simulink model "xaui_monitor_test"  (Simulink 7.0)
settings: Solver=ode45  StartTime=0.0  StopTime=100  RelTol=1e-3
libraries: xbsIndex_r4 x34, casper_library_misc x5
settings Model: Creator=mdexter  LastModifiedBy=mdexter

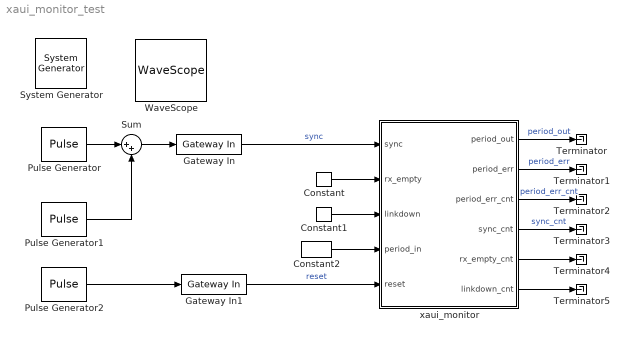
== system xaui_monitor_test ==
  " System Generator" : xbsIndex_r4/ System Generator  Tag=genX  SystemSampleTime=-1  xilinxfamily=Virtex4  part=xc4vsx35  speed=-10  package=ff668  synthesis_tool=XST  clock_wrapper=Clock Enables  directory=./netlist  testbench=off  simulink_period=1  sysclk_period=100  dcm_input_clock_period=100  incr_netlist=off  trim_vbits=Everywhere in SubSystem  dbl_ovrd=According to Block Masks  core_generation=According to Block Masks  run_coregen=off  deprecated_control=off  eval_field=0  block_type=sysgen
      settings: block_version=10.1.3
  Constant : xbsIndex_r4/Constant  arith_type=Boolean  const=0  n_bits=16  bin_pt=14  explicit_period=on  period=1  equ=P=C  opselect=C  inp2=PCIN>>17  opr=+  inp1=P  carry=CIN  dbl_ovrd=off  block_type=constant
  Constant1 : xbsIndex_r4/Constant  arith_type=Boolean  const=0  n_bits=16  bin_pt=14  explicit_period=on  period=1  equ=P=C  opselect=C  inp2=PCIN>>17  opr=+  inp1=P  carry=CIN  dbl_ovrd=off  block_type=constant
  Constant2 : xbsIndex_r4/Constant  arith_type=Unsigned  const=10  n_bits=32  bin_pt=0  explicit_period=on  period=1  equ=P=C  opselect=C  inp2=PCIN>>17  opr=+  inp1=P  carry=CIN  dbl_ovrd=off  block_type=constant
  Gateway In : xbsIndex_r4/Gateway In  arith_type=Boolean  n_bits=16  bin_pt=14  quantization="Round  (unbiased: +/- Inf)"  overflow=Saturate  period=1  dbl_ovrd=off  timing_constraint=None  locs_specified=off  LOCs={}  block_type=gatewayin
      settings: infoedit="Gateway in block.  Converts inputs of type Simulink integer, double and fixed point to  Xilinx fixed point type.<P><P>Hardware notes:  In hardware these blocks become top level input ports."  block_version=10.1.3
  Gateway In1 : xbsIndex_r4/Gateway In  arith_type=Boolean  n_bits=16  bin_pt=14  quantization="Round  (unbiased: +/- Inf)"  overflow=Saturate  period=1  dbl_ovrd=off  timing_constraint=None  locs_specified=off  LOCs={}  block_type=gatewayin
      settings: infoedit="Gateway in block.  Converts inputs of type Simulink integer, double and fixed point to  Xilinx fixed point type.<P><P>Hardware notes:  In hardware these blocks become top level input ports."  block_version=10.1.3
  Pulse Generator : DiscretePulseGenerator  Period=10  VectorParams1D=off
  Pulse Generator1 : DiscretePulseGenerator  Period=1e3  PhaseDelay=34  VectorParams1D=off
  Pulse Generator2 : DiscretePulseGenerator  Period=1e3  PhaseDelay=49  VectorParams1D=off
  Sum : Sum  Inputs=|++  OutDataType=sfix(16)  OutScaling=2^0
  Terminator{,1..5} (6 alike) : Terminator
  WaveScope : xbsIndex_r4/WaveScope  block_type=wavescope
      settings: block_version=10.1.3
  xaui_monitor : Subsystem
  wires:
  Gateway In/1 -> xaui_monitor/1(sync)  "sync"
  Constant/1 -> xaui_monitor/2(rx_empty)
  Constant1/1 -> xaui_monitor/3(linkdown)
  Constant2/1 -> xaui_monitor/4(period_in)
  Gateway In1/1 -> xaui_monitor/5(reset)  "reset"
  xaui_monitor/1(period_out) -> Terminator/1  "period_out"
  xaui_monitor/2(period_err) -> Terminator1/1  "period_err"
  xaui_monitor/3(period_err_cnt) -> Terminator2/1  "period_err_cnt"
  xaui_monitor/4(sync_cnt) -> Terminator3/1  "sync_cnt"
  xaui_monitor/5(rx_empty_cnt) -> Terminator4/1
  xaui_monitor/6(linkdown_cnt) -> Terminator5/1
  Pulse Generator/1 -> Sum/1
  Sum/1 -> Gateway In/1
  Pulse Generator1/1 -> Sum/2
  Pulse Generator2/1 -> Gateway In1/1

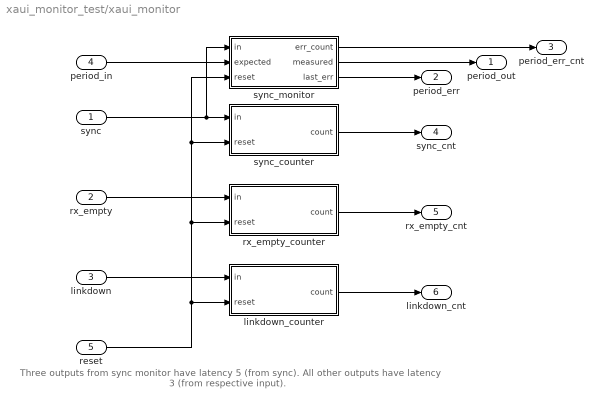
== system xaui_monitor_test/xaui_monitor ==
  note: Three outputs from sync monitor have latency 5 (from sync).
      | All other outputs have latency 3 (from respective input).
  sync : Inport
  rx_empty : Inport  Port=2
  linkdown : Inport  Port=3
  period_in : Inport  Port=4
  reset : Inport  Port=5
  linkdown_counter : Subsystem
      settings: AttributesFormatString=rising
  rx_empty_counter : Subsystem
      settings: AttributesFormatString=rising
  sync_counter : Subsystem
      settings: AttributesFormatString=rising
  sync_monitor : Subsystem
  period_out : Outport
  period_err : Outport  Port=2
  period_err_cnt : Outport  Port=3
  sync_cnt : Outport  Port=4
  rx_empty_cnt : Outport  Port=5
  linkdown_cnt : Outport  Port=6
  wires:
  sync/1 -> sync_monitor/1(in), sync_counter/1(in)
  sync_monitor/1(err_count) -> period_err_cnt/1
  period_in/1 -> sync_monitor/2(expected)
  sync_monitor/2(measured) -> period_out/1
  sync_monitor/3(last_err) -> period_err/1
  sync_counter/1(count) -> sync_cnt/1
  rx_empty/1 -> rx_empty_counter/1(in)
  rx_empty_counter/1(count) -> rx_empty_cnt/1
  linkdown/1 -> linkdown_counter/1(in)
  linkdown_counter/1(count) -> linkdown_cnt/1
  reset/1 -> sync_monitor/3(reset), sync_counter/2(reset), rx_empty_counter/2(reset), linkdown_counter/2(reset)

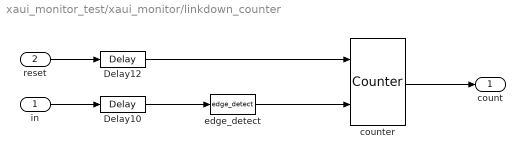
== system xaui_monitor_test/xaui_monitor/linkdown_counter ==
  in : Inport  OutDataType=sfix(16)  OutScaling=2^0
  reset : Inport  Port=2  OutDataType=sfix(16)  OutScaling=2^0
  Delay10 : xbsIndex_r4/Delay  en=off  latency=1  dbl_ovrd=off  reg_retiming=off  block_type=delay
      settings: xl_area=[0, 0, 0, 0, 0, 0, 0]
  Delay12 : xbsIndex_r4/Delay  en=off  latency=1  dbl_ovrd=off  reg_retiming=off  block_type=delay
      settings: xl_area=[0, 0, 0, 0, 0, 0, 0]
  counter : xbsIndex_r4/Counter  cnt_type=Free Running  cnt_to=Inf  operation=Up  start_count=0  cnt_by_val=1  arith_type=Unsigned  n_bits=32  bin_pt=0  load_pin=off  rst=on  en=on  explicit_period=off  period=1  dbl_ovrd=off  use_behavioral_HDL=on  use_rpm=on  implementation=Fabric  block_type=counter
      settings: xl_area=[0, 0, 0, 0, 0, 0, 0]
  edge_detect : casper_library_misc/edge_detect  SystemSampleTime=-1  edge=Rising  polarity=Active High  x_in=[0 0.08 0.08 0.16 0.16 0.24 0.24 0.32 0.32 0.4]  y_in="[-1 -1  1  1  1  1  1  1  1  1]"  x_out=[0.6 0.68 0.68 0.76 0.76 0.84 0.84 0.92 0.92 1]  y_out="[-1 -1  1  1 -1 -1 -1 -1 -1 -1]"
  count : Outport  OutDataType=sfix(16)  OutScaling=2^0
  wires:
  in/1 -> Delay10/1
  reset/1 -> Delay12/1
  Delay10/1 -> edge_detect/1
  Delay12/1 -> counter/1
  counter/1 -> count/1
  edge_detect/1 -> counter/2

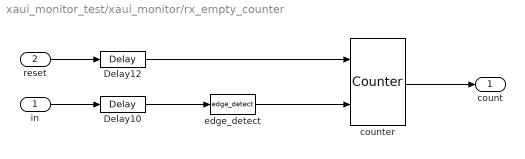
== system xaui_monitor_test/xaui_monitor/rx_empty_counter ==
  in : Inport  OutDataType=sfix(16)  OutScaling=2^0
  reset : Inport  Port=2  OutDataType=sfix(16)  OutScaling=2^0
  Delay10 : xbsIndex_r4/Delay  en=off  latency=1  dbl_ovrd=off  reg_retiming=off  block_type=delay
      settings: xl_area=[0, 0, 0, 0, 0, 0, 0]
  Delay12 : xbsIndex_r4/Delay  en=off  latency=1  dbl_ovrd=off  reg_retiming=off  block_type=delay
      settings: xl_area=[0, 0, 0, 0, 0, 0, 0]
  counter : xbsIndex_r4/Counter  cnt_type=Free Running  cnt_to=Inf  operation=Up  start_count=0  cnt_by_val=1  arith_type=Unsigned  n_bits=32  bin_pt=0  load_pin=off  rst=on  en=on  explicit_period=off  period=1  dbl_ovrd=off  use_behavioral_HDL=on  use_rpm=on  implementation=Fabric  block_type=counter
      settings: xl_area=[0, 0, 0, 0, 0, 0, 0]
  edge_detect : casper_library_misc/edge_detect  SystemSampleTime=-1  edge=Rising  polarity=Active High  x_in=[0 0.08 0.08 0.16 0.16 0.24 0.24 0.32 0.32 0.4]  y_in="[-1 -1  1  1  1  1  1  1  1  1]"  x_out=[0.6 0.68 0.68 0.76 0.76 0.84 0.84 0.92 0.92 1]  y_out="[-1 -1  1  1 -1 -1 -1 -1 -1 -1]"
  count : Outport  OutDataType=sfix(16)  OutScaling=2^0
  wires:
  in/1 -> Delay10/1
  reset/1 -> Delay12/1
  Delay10/1 -> edge_detect/1
  Delay12/1 -> counter/1
  counter/1 -> count/1
  edge_detect/1 -> counter/2

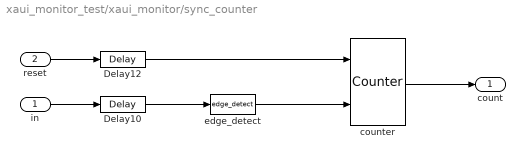
== system xaui_monitor_test/xaui_monitor/sync_counter ==
  in : Inport  OutDataType=sfix(16)  OutScaling=2^0
  reset : Inport  Port=2  OutDataType=sfix(16)  OutScaling=2^0
  Delay10 : xbsIndex_r4/Delay  en=off  latency=1  dbl_ovrd=off  reg_retiming=off  block_type=delay
      settings: xl_area=[0, 0, 0, 0, 0, 0, 0]
  Delay12 : xbsIndex_r4/Delay  en=off  latency=1  dbl_ovrd=off  reg_retiming=off  block_type=delay
      settings: xl_area=[0, 0, 0, 0, 0, 0, 0]
  counter : xbsIndex_r4/Counter  cnt_type=Free Running  cnt_to=Inf  operation=Up  start_count=0  cnt_by_val=1  arith_type=Unsigned  n_bits=32  bin_pt=0  load_pin=off  rst=on  en=on  explicit_period=off  period=1  dbl_ovrd=off  use_behavioral_HDL=on  use_rpm=on  implementation=Fabric  block_type=counter
      settings: xl_area=[0, 0, 0, 0, 0, 0, 0]
  edge_detect : casper_library_misc/edge_detect  SystemSampleTime=-1  edge=Rising  polarity=Active High  x_in=[0 0.08 0.08 0.16 0.16 0.24 0.24 0.32 0.32 0.4]  y_in="[-1 -1  1  1  1  1  1  1  1  1]"  x_out=[0.6 0.68 0.68 0.76 0.76 0.84 0.84 0.92 0.92 1]  y_out="[-1 -1  1  1 -1 -1 -1 -1 -1 -1]"
  count : Outport  OutDataType=sfix(16)  OutScaling=2^0
  wires:
  in/1 -> Delay10/1
  reset/1 -> Delay12/1
  Delay10/1 -> edge_detect/1
  Delay12/1 -> counter/1
  counter/1 -> count/1
  edge_detect/1 -> counter/2

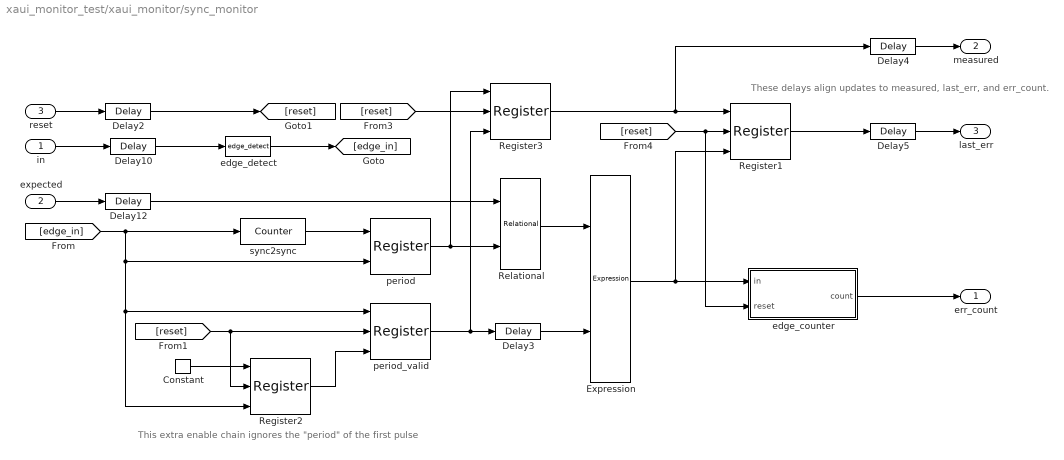
== system xaui_monitor_test/xaui_monitor/sync_monitor ==
  note: This extra enable chain ignores the "period" of the first pulse
  note: These delays align updates to
      | measured, last_err, and err_count.
  in : Inport
  expected : Inport  Port=2
  reset : Inport  Port=3
  Constant : xbsIndex_r4/Constant  arith_type=Boolean  const=1  n_bits=16  bin_pt=14  explicit_period=on  period=1  equ=P=C  opselect=C  inp2=PCIN>>17  opr=+  inp1=P  carry=CIN  dbl_ovrd=off  block_type=constant
  Delay{2..3,5,10,12} (5 alike) : xbsIndex_r4/Delay  en=off  latency=1  dbl_ovrd=off  reg_retiming=off  block_type=delay
      settings: xl_area=[0, 0, 0, 0, 0, 0, 0]
  Delay4 : xbsIndex_r4/Delay  en=off  latency=2  dbl_ovrd=off  reg_retiming=off  block_type=delay
      settings: xl_area=[0, 0, 0, 0, 0, 0, 0]
  Expression : xbsIndex_r4/Expression  expression=a & b  align_bp=on  en=off  latency=0  precision=Full  arith_type=Unsigned  n_bits=16  bin_pt=0  dbl_ovrd=off  block_type=expr
      settings: block_version=10.1.3
  Register1 : xbsIndex_r4/Register  init=0  rst=on  en=on  dbl_ovrd=off  block_type=register
  Register2 : xbsIndex_r4/Register  init=0  rst=on  en=on  dbl_ovrd=off  block_type=register
  Register3 : xbsIndex_r4/Register  init=0  rst=on  en=on  dbl_ovrd=off  block_type=register
  Relational : xbsIndex_r4/Relational  mode=a!=b  en=off  latency=1  dbl_ovrd=off  block_type=relational
      settings: block_version=10.1.3
  edge_counter : Subsystem
      settings: AttributesFormatString=rising
  edge_detect : casper_library_misc/edge_detect  SystemSampleTime=-1  edge=Rising  polarity=Active High  x_in=[0 0.08 0.08 0.16 0.16 0.24 0.24 0.32 0.32 0.4]  y_in="[-1 -1  1  1  1  1  1  1  1  1]"  x_out=[0.6 0.68 0.68 0.76 0.76 0.84 0.84 0.92 0.92 1]  y_out="[-1 -1  1  1 -1 -1 -1 -1 -1 -1]"
  period : xbsIndex_r4/Register  init=0  rst=off  en=on  dbl_ovrd=off  block_type=register
  period_valid : xbsIndex_r4/Register  init=0  rst=on  en=on  dbl_ovrd=off  block_type=register
  sync2sync : xbsIndex_r4/Counter  cnt_type=Free Running  cnt_to=Inf  operation=Up  start_count=1  cnt_by_val=1  arith_type=Unsigned  n_bits=32  bin_pt=0  load_pin=off  rst=on  en=off  explicit_period=off  period=1  dbl_ovrd=off  use_behavioral_HDL=on  use_rpm=on  implementation=Fabric  block_type=counter
      settings: xl_area=[0, 0, 0, 0, 0, 0, 0]
  err_count : Outport  OutDataType=sfix(16)  OutScaling=2^0
  measured : Outport  Port=2  OutDataType=sfix(16)  OutScaling=2^0
  last_err : Outport  Port=3  OutDataType=sfix(16)  OutScaling=2^0
  wires:
  sync2sync/1 -> period/1
  [edge_in] -> sync2sync/1, period/2, period_valid/1, Register2/3
  Relational/1 -> Expression/1
  Delay3/1 -> Expression/2
  Expression/1 -> edge_counter/1(in), Register1/3
  period/1 -> Relational/2, Register3/1
  expected/1 -> Delay12/1
  reset/1 -> Delay2/1
  edge_counter/1(count) -> err_count/1
  Register1/1 -> Delay5/1
  Register3/1 -> Register1/1, Delay4/1
  Delay10/1 -> edge_detect/1
  in/1 -> Delay10/1
  Delay12/1 -> Relational/1
  edge_detect/1 -> [edge_in]
  Delay2/1 -> [reset]
  Constant/1 -> Register2/1
  period_valid/1 -> Delay3/1, Register3/3
  Delay4/1 -> measured/1
  Delay5/1 -> last_err/1
  Register2/1 -> period_valid/3
  [reset] -> period_valid/2, Register2/2
  [reset] -> Register3/2
  [reset] -> Register1/2, edge_counter/2(reset)

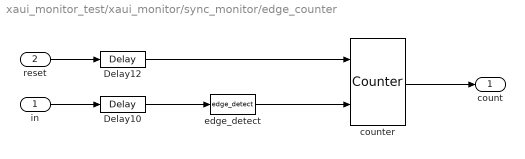
== system xaui_monitor_test/xaui_monitor/sync_monitor/edge_counter ==
  in : Inport  OutDataType=sfix(16)  OutScaling=2^0
  reset : Inport  Port=2  OutDataType=sfix(16)  OutScaling=2^0
  Delay10 : xbsIndex_r4/Delay  en=off  latency=1  dbl_ovrd=off  reg_retiming=off  block_type=delay
      settings: xl_area=[0, 0, 0, 0, 0, 0, 0]
  Delay12 : xbsIndex_r4/Delay  en=off  latency=1  dbl_ovrd=off  reg_retiming=off  block_type=delay
      settings: xl_area=[0, 0, 0, 0, 0, 0, 0]
  counter : xbsIndex_r4/Counter  cnt_type=Free Running  cnt_to=Inf  operation=Up  start_count=0  cnt_by_val=1  arith_type=Unsigned  n_bits=32  bin_pt=0  load_pin=off  rst=on  en=on  explicit_period=off  period=1  dbl_ovrd=off  use_behavioral_HDL=on  use_rpm=on  implementation=Fabric  block_type=counter
      settings: xl_area=[0, 0, 0, 0, 0, 0, 0]
  edge_detect : casper_library_misc/edge_detect  SystemSampleTime=-1  edge=Rising  polarity=Active High  x_in=[0 0.08 0.08 0.16 0.16 0.24 0.24 0.32 0.32 0.4]  y_in="[-1 -1  1  1  1  1  1  1  1  1]"  x_out=[0.6 0.68 0.68 0.76 0.76 0.84 0.84 0.92 0.92 1]  y_out="[-1 -1  1  1 -1 -1 -1 -1 -1 -1]"
  count : Outport  OutDataType=sfix(16)  OutScaling=2^0
  wires:
  in/1 -> Delay10/1
  reset/1 -> Delay12/1
  Delay10/1 -> edge_detect/1
  Delay12/1 -> counter/1
  counter/1 -> count/1
  edge_detect/1 -> counter/2
